simulink model "BAES_RAGUSANTE_Block_Diagram_Algebra_NUMBER1_ORIGINAL"  (R2023b)
settings: Solver=VariableStepAuto  StartTime=0.0  StopTime=20  RelTol=1e-3
values from neighbouring files (symbols this model uses):
  G1_den = [1 0 0]    [BAES_RAGUSANTE_Block_Diagram_Algebra_NUMBER1_ORIGINAL.m]    (also in BAES_RAGUSANTE_Block_Diagram_Algebra_NUMBER1_REDUCED.m; LOISAGA_GARCIA_BlockDiagramAlgebra_Problem2.m)
  G1_num = [0 1]    [BAES_RAGUSANTE_Block_Diagram_Algebra_NUMBER1_ORIGINAL.m]    (also in BAES_RAGUSANTE_Block_Diagram_Algebra_NUMBER1_REDUCED.m; LOISAGA_GARCIA_BlockDiagramAlgebra_Problem2.m = 1)
  G2_den = [1 1]    [BAES_RAGUSANTE_Block_Diagram_Algebra_NUMBER1_ORIGINAL.m]    (also in BAES_RAGUSANTE_Block_Diagram_Algebra_NUMBER1_REDUCED.m; LOISAGA_GARCIA_BlockDiagramAlgebra_Problem2.m)
  G2_num = [0 1]    [BAES_RAGUSANTE_Block_Diagram_Algebra_NUMBER1_ORIGINAL.m]    (also in BAES_RAGUSANTE_Block_Diagram_Algebra_NUMBER1_REDUCED.m; LOISAGA_GARCIA_BlockDiagramAlgebra_Problem2.m = 1)
  G3_den = [1 0]    [BAES_RAGUSANTE_Block_Diagram_Algebra_NUMBER1_ORIGINAL.m]    (also in BAES_RAGUSANTE_Block_Diagram_Algebra_NUMBER1_REDUCED.m; LOISAGA_GARCIA_BlockDiagramAlgebra_Problem2.m)
  G3_num = [0 1]    [BAES_RAGUSANTE_Block_Diagram_Algebra_NUMBER1_ORIGINAL.m]    (also in BAES_RAGUSANTE_Block_Diagram_Algebra_NUMBER1_REDUCED.m; LOISAGA_GARCIA_BlockDiagramAlgebra_Problem2.m = 1)
  H1_den = [1 0]    [BAES_RAGUSANTE_Block_Diagram_Algebra_NUMBER1_ORIGINAL.m]    (also in BAES_RAGUSANTE_Block_Diagram_Algebra_NUMBER1_REDUCED.m; LOISAGA_GARCIA_BlockDiagramAlgebra_Problem2.m)
  H1_num = [0 1]    [BAES_RAGUSANTE_Block_Diagram_Algebra_NUMBER1_ORIGINAL.m]    (also in BAES_RAGUSANTE_Block_Diagram_Algebra_NUMBER1_REDUCED.m; LOISAGA_GARCIA_BlockDiagramAlgebra_Problem2.m = 1)
  H2_den = [1 -1]    [BAES_RAGUSANTE_Block_Diagram_Algebra_NUMBER1_ORIGINAL.m]    (also in BAES_RAGUSANTE_Block_Diagram_Algebra_NUMBER1_REDUCED.m; LOISAGA_GARCIA_BlockDiagramAlgebra_Problem2.m)
  H2_num = [0 1]    [BAES_RAGUSANTE_Block_Diagram_Algebra_NUMBER1_ORIGINAL.m]    (also in BAES_RAGUSANTE_Block_Diagram_Algebra_NUMBER1_REDUCED.m; LOISAGA_GARCIA_BlockDiagramAlgebra_Problem2.m = 1)
  H3_den = [1 -2]    [BAES_RAGUSANTE_Block_Diagram_Algebra_NUMBER1_ORIGINAL.m]    (also in BAES_RAGUSANTE_Block_Diagram_Algebra_NUMBER1_REDUCED.m; LOISAGA_GARCIA_BlockDiagramAlgebra_Problem2.m)
  H3_num = [0 1]    [BAES_RAGUSANTE_Block_Diagram_Algebra_NUMBER1_ORIGINAL.m]    (also in BAES_RAGUSANTE_Block_Diagram_Algebra_NUMBER1_REDUCED.m; LOISAGA_GARCIA_BlockDiagramAlgebra_Problem2.m = 1)
settings Model: Creator=Mary Belle Baes  LastModifiedBy=Mary Belle Baes

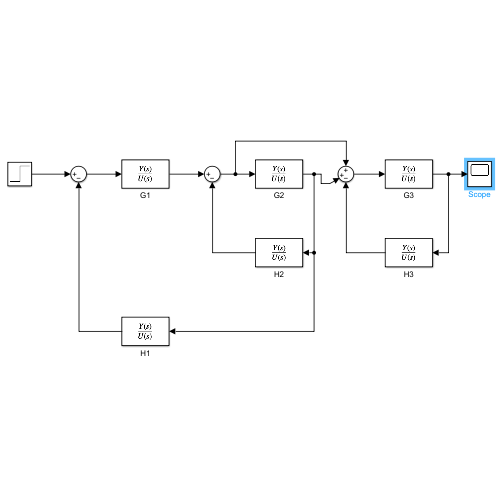
[thumbnail: Simulink's stored preview of the top-level diagram]
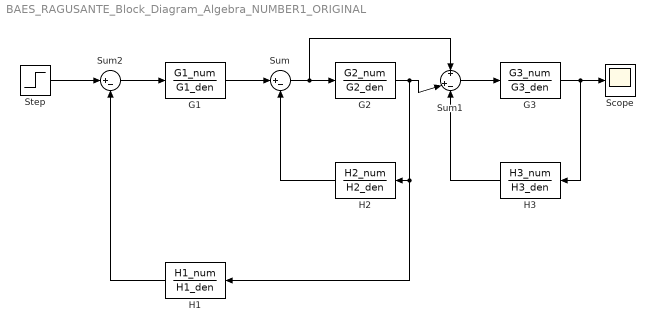
== system BAES_RAGUSANTE_Block_Diagram_Algebra_NUMBER1_ORIGINAL ==
  G1 : TransferFcn  Numerator=G1_num  Denominator=G1_den
  G2 : TransferFcn  Numerator=G2_num  Denominator=G2_den
  G3 : TransferFcn  Numerator=G3_num  Denominator=G3_den
  H1 : TransferFcn  Numerator=H1_num  Denominator=H1_den
  H2 : TransferFcn  Numerator=H2_num  Denominator=H2_den
  H3 : TransferFcn  Numerator=H3_num  Denominator=H3_den
  Scope : Scope
  Step : Step  Time=0  SampleTime=0
  Sum : Sum  Inputs=|+-
  Sum1 : Sum  Inputs=+|+-
  Sum2 : Sum  Inputs=|+-
  wires:
  Step/1 -> Sum2/1
  Sum2/1 -> G1/1
  G1/1 -> Sum/1
  Sum/1 -> Sum1/1, G2/1
  G3/1 -> H3/1, Scope/1
  Sum1/1 -> G3/1
  H1/1 -> Sum2/2
  H3/1 -> Sum1/3
  H2/1 -> Sum/2
  G2/1 -> H1/1, H2/1, Sum1/2
